simulink model "bldc_cImpl"  (R2018a)
settings: Solver=FixedStepDiscrete  StartTime=0.0  StopTime=5  FixedStep=Ts  RelTol=1e-3  EnableMultiTasking=on
undefined symbols (not defined in the file): fsw, Imax, Ki_id, Ki_iq, Kp_id, Kp_iq, Ld, p, Pmax, psim, sigbuilder_block, Tmax, Ts, Tsi, V1, Vnom, wbase
libraries: nesl_utility x12, fl_lib x11, pe_lib x5, pePwmGenerator x3, simulink_extras x1
Description:
  | IPMSM Torque Control in an Axle-Drive EV
  | 
  | Copyright 2017 The MathWorks, Inc.
settings Model: Creator=The MathWorks, Inc.  LastModifiedBy=Acer
settings SolverCC: AutoInsertRateTranBlk=on
settings DataIOCC: MaxDataPoints=510000  SignalLoggingName=logsout_pe_ipmsm_torque_control_ev_axle
settings OptimizationCC: LifeSpan=inf
settings DebuggingCC: UnderspecifiedInitializationDetection=Classic  MergeDetectMultiDrivingBlocksExec=none  SFUnexpectedBacktrackingDiag=warning  SFNoUnconditionalDefaultTransitionDiag=warning  SFExecutionAtInitializationDiag=none
settings CodeAppCC: StateflowObjectComments=on
settings GRTTargetCC: TargetLangStandard=C89/C90 (ANSI)  GeneratePreprocessorConditionals=Disable all
settings ConfigComp: CovMetricSettings=dw  CovHtmlReporting=on  CovSaveCumulativeToWorkspaceVar=on  CovSaveSingleToWorkspaceVar=on  CovExternalEMLEnable=off
settings SimscapeCC: SimscapeNormalizeSystem=off  SimscapeLogType=all  SimscapeLogSimulationStatistics=on  SimscapeLogName=simlog_pe_ipmsm_torque_control_ev_axle  SimscapeLogDataHistory=510000

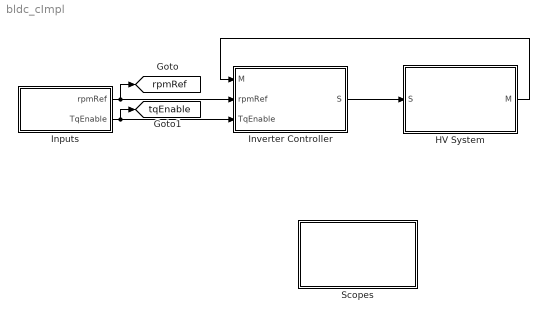
== system bldc_cImpl ==
  HV System : Subsystem
  Inputs : Subsystem  Tag=STV Subsys  LoadFcn=sigbuilder_block('load');  StartFcn=sigbuilder_block('start');  StopFcn=sigbuilder_block('stop');  ClipboardFcn=sigbuilder_block('clipboard');  mask(Sigbuilder block){tuvar=[0:10]}
      mask help: Simulink:masks:SigbuilderBlock_MD
      mask init:
      | if ~strcmp(get_param(bdroot(gcbh),'SimulationStatus'),'stopped') tuvar = sigbuilder_block('maskInit'); end
      settings: CopyFcn=sigbuilder_block('copy');  DeleteFcn=sigbuilder_block('delete');  ModelCloseFcn=sigbuilder_block('modelClose');  PreSaveFcn=sigbuilder_block('preSave');  PauseFcn=sigbuilder_block('pause');  ContinueFcn=sigbuilder_block('continue');  NameChangeFcn=sigbuilder_block('namechange');  OpenFcn=sigbuilder_block('open',[627 127.5 1012.5 512.25 ]);  CloseFcn=sigbuilder_block('close');
      mask Display: plot(0, 0, 100, 100,[2, 2, 32, 32, 2], [68, 8, 8, 68, 68],[32, 2], [38, 38], [32, 19, 2],[53, 60, 44], [32, 17, 17, 2],[16, 16, 31, 31]);txt = getActiveGroup(gcbh);text(2, 100, txt,'verticalAlignment', 'top');
  Inverter Controller : Subsystem
  Scopes : Subsystem
  tag scope: rpmRef=global, tqEnable=global
  wires:
  Inverter Controller/1(S) -> HV System/1(S)
  HV System/1(M) -> Inverter Controller/1(M)
  Inputs/1(rpmRef) -> Inverter Controller/2(rpmRef), [rpmRef]
  Inputs/2(TqEnable) -> [tqEnable], Inverter Controller/3(TqEnable)

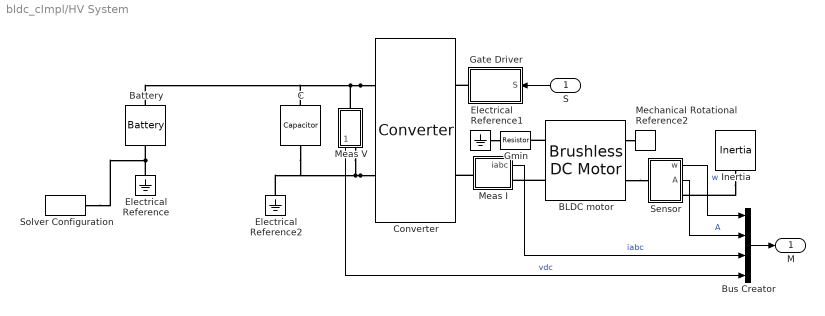
== system bldc_cImpl/HV System ==
  S : Inport
  BLDC motor : pe_lib/Machines/Permanent Magnet Rotor/Brushless DC Motor  rotor_param=1  pm_flux_linkage=psim Wb  theta_constant=pi / 12 rad  emf_max=9.6 V  DphiDtheta_tab=[0, -.1528, -.1528, .1528, .1528, 0] Wb/rad  back_emf_tab=[0, -9.6, -9.6, 9.6, 9.6, 0] V  rotor_angle_tab=[0, 7.5, 22.5, 37.5, 52.5, 60] deg  w_meas=600 rpm  nPolePairs=p  stator_param=1  Ld=Ld H  Lq=Lq H  L0=L0 H  Ls=0.0002 H  Lm=0 H  Ms=0.00002 H  Rs=Rs Ohm  zero_sequence=pe.enum.park.zerosequence.exclude  J=0 kg*m^2  lam=0 N*m/(rad/s)  axes_param=1  i_d_specify=off  i_d_priority=None  i_d=0 A  i_d_nominal_specify=off  i_d_nominal_unit=A  i_d_nominal_value=1  i_q_specify=off  i_q_priority=None  i_q=0 A  i_q_nominal_specify=off  i_q_nominal_unit=A  i_q_nominal_value=1  torque_specify=off  torque_priority=None  torque=0 N*m  torque_nominal_specify=off  torque_nominal_unit=N*m  torque_nominal_value=1  angular_velocity_specify=on  angular_velocity_priority=High  angular_velocity=0 rpm  angular_velocity_nominal_specify=off  angular_velocity_nominal_unit=rpm  angular_velocity_nominal_value=1  angular_position_specify=off  angular_position_priority=High  angular_position=0 deg  angular_position_nominal_specify=off  angular_position_nominal_unit=deg  angular_position_nominal_value=1
      settings: SourceProductName=Simscape Power Systems  SourceProductBaseCode=PS
  Battery : pe_lib/Sources/Battery  Vnom=Vnom V  R1=0.001 Ohm  prm_AH=1  AH=15000 hr*A  V1=V1 V  AH1=10000 hr*A  prm_R2=1  R2=2000 Ohm  prm_dyn=1  Rp1=0.005 Ohm  tau1=30 s  Rp2=0.005 Ohm  tau2=30 s  prm_fade=1  N_fade=100  AH_fade=45 hr*A  R1_fade=2.02 Ohm  V1_fade=10.35 V  i_specify=off  i_priority=None  i=0 A  i_nominal_specify=off  i_nominal_unit=A  i_nominal_value=1  v_specify=off  v_priority=None  v=0 V  v_nominal_specify=off  v_nominal_unit=V  v_nominal_value=1  charge_specify=on  charge_priority=High  charge=14000 hr*A  charge_nominal_specify=off  charge_nominal_unit=hr*A  charge_nominal_value=1  num_cycles_specify=off  num_cycles_priority=High  num_cycles=0  num_cycles_nominal_specify=off  num_cycles_nominal_unit=1  num_cycles_nominal_value=1  thermal_mass=30000 J/K  Tmeas=298.15 K  Vnom_T2=12 V  R1_T2=2.2 Ohm  V1_T2=11.4 V  R2_T2=2200 Ohm  Rp1_T2=0.005 Ohm  tau1_T2=30 s  Rp2_T2=0.005 Ohm  tau2_T2=30 s  Tmeas2=273.15 K  temperature_specify=off  temperature_priority=High  temperature=298.15 K  temperature_nominal_specify=off  temperature_nominal_unit=K  temperature_nominal_value=1
      settings: SourceProductName=Simscape Power Systems  SourceProductBaseCode=PS
  Bus Creator : BusCreator  Inputs=4
  C : fl_lib/Electrical/Electrical Elements/Capacitor  c=Cdc F  r=1e-6 Ohm  g=0 1/Ohm  i_specify=off  i_priority=None  i=0 A  i_nominal_specify=off  i_nominal_unit=A  i_nominal_value=1  v_specify=off  v_priority=None  v=0 V  v_nominal_specify=off  v_nominal_unit=V  v_nominal_value=1  vc_specify=off  vc_priority=High  vc=0 V  vc_nominal_specify=off  vc_nominal_unit=V  vc_nominal_value=1
      settings: SourceProductName=Foundation Library
  Converter : pe_lib/Semiconductors/Converter  device_type=3  Vf=0.8 V  Ron=0.001 Ohm  Rds=0.001 Ohm  Goff=1e-5 1/Ohm  Vth=0.5 V  Vgt=1 V  Vgt_off=-1 V  Ih=1 A  diode_param=2  diode_Vf=0.8 V  diode_Ron=0.001 Ohm  diode_Goff=1e-5 1/Ohm  diode_C=50 nF  diode_iRM=-235 A  diode_iF=300 A  diode_idot=-50 A/us  diode_trr_param=1  diode_trr_factor=3  diode_trr=15 us  diode_Qrr=1.5e+3 s*uA  snubber_type=0  Rs=0.1 Ohm  Cs=1e-7 F
      settings: SourceProductName=Simscape Power Systems  SourceProductBaseCode=PS
  Electrical Reference : fl_lib/Electrical/Electrical Elements/Electrical Reference
      settings: SourceProductName=Foundation Library
  Electrical Reference1 : fl_lib/Electrical/Electrical Elements/Electrical Reference
      settings: SourceProductName=Foundation Library
  Electrical Reference2 : fl_lib/Electrical/Electrical Elements/Electrical Reference
      settings: SourceProductName=Foundation Library
  Gate Driver : Subsystem
  Gmin : fl_lib/Electrical/Electrical Elements/Resistor  R=1e9 Ohm  i_specify=off  i_priority=High  i=0 A  i_nominal_specify=off  i_nominal_unit=A  i_nominal_value=1  v_specify=off  v_priority=High  v=0 V  v_nominal_specify=off  v_nominal_unit=V  v_nominal_value=1
      settings: SourceProductName=Foundation Library
  Inertia : fl_lib/Mechanical/Rotational Elements/Inertia  inertia=Jm kg*m^2  w_specify=off  w_priority=High  w=0 rad/s  w_nominal_specify=off  w_nominal_unit=rad/s  w_nominal_value=1  t_specify=off  t_priority=None  t=0 N*m  t_nominal_specify=off  t_nominal_unit=N*m  t_nominal_value=1
      settings: SourceProductName=Foundation Library
  Meas I : Subsystem
      mask Display: %disp('iABC');
  Meas V : Subsystem
  Mechanical Rotational Reference2 : fl_lib/Mechanical/Rotational Elements/Mechanical Rotational Reference
      settings: SourceProductName=Foundation Library
  Sensor : Subsystem
  Solver Configuration : nesl_utility/Solver Configuration  PhysicalDomain=network_engine_domain  SubClassName=solver  LeftPortType=input  RightPortType=generic  Tones=[]  Harmonics=[]  SimulateNoise=off  Profile=off  UseLocalSampling=off  EnableSwitchedLinearOptims=on  FrequencyDomain=off  UseCCode=off  RelTol=0.001  AbsTol=1e-06  MinStep=1e-09  ToWorkspace=off  RevertToSquareIcSolve=off  NumHomotopyIterations=100  PhasorMode=off  PhasorModeNumHarmonics=1  DoDC=off  ResidualTolerance=1e-9  UseLocalSolver=on  LocalSolverChoice=NE_BACKWARD_EULER_ADVANCER  LocalSolverSampleTime=Ts  DoFixedCost=on  MaxNonlinIter=4  MaxModeIter=2  LinearAlgebra=Sparse  EquationFormulation=NE_TIME_EF  DelaysMemoryBudget=1024  AutomaticFiltering=on  FilteringTimeConstant=0.001
  M : Outport
  wires:
  Meas V/1(Vdc) -> Bus Creator/4  "vdc"
  Sensor/2(A) -> Bus Creator/2  "A"
  Bus Creator/1 -> M/1
  Sensor/1(w) -> Bus Creator/1  "w"
  Meas I/1(iabc) -> Bus Creator/3  "iabc"
  S/1 -> Gate Driver/1(S)
  connections:
  Converter/RConn2 -- Electrical Reference2/LConn1 -- C/RConn1 -- Meas V/RConn1
  Converter/RConn1 -- Battery/LConn1 -- C/LConn1 -- Meas V/LConn1
  Inertia/LConn1 -- Sensor/RConn1
  BLDC motor/RConn2 -- Mechanical Rotational Reference2/LConn1
  BLDC motor/LConn1 -- Meas I/RConn1
  Gate Driver/RConn1 -- Converter/LConn1
  Meas I/LConn1 -- Converter/LConn2
  Electrical Reference1/LConn1 -- Gmin/LConn1
  BLDC motor/RConn1 -- Sensor/LConn1
  BLDC motor/LConn2 -- Gmin/RConn1
  Battery/RConn1 -- Electrical Reference/LConn1 -- Solver Configuration/RConn1

== system bldc_cImpl/Inputs ==
  Demux : Demux  Tag=STV Demux  Outputs=2
  FromWs : FromWorkspace  Tag=STV FromWs  VariableName=tuvar  SampleTime=0
      SigBuilderData=|
      | common.afterFinalStr = 'Extrapolate'
      | common.sampleTime = 0
      | dataSet.timeRange = [0 15]
      | dataSet.name = 'Default'
      | sbobj.Groups.Name = 'Default'
      | sbobj.Groups.Signals(1).Name = 'rpmRef'
      | sbobj.Groups.Signals(1).XData = [0 0.7 0.7 2 2 3.12 3.5 4 4.5 15]
      | sbobj.Groups.Signals(1).YData = [0 0 1500 1500 0 0 -1000 -1000 0 0]
      | sbobj.Groups.Signals(2).Name = 'TqEnable'
      | sbobj.Groups.Signals(2).XData = [0 15]
      | sbobj.Groups.Signals(2).YData = [1 1]
      | sbobj.Groups.TimeRange = [0 15]
  rpmRef : Outport  Tag=STV Outport
  TqEnable : Outport  Tag=STV Outport  Port=2
  wires:
  FromWs/1 -> Demux/1
  Demux/1 -> rpmRef/1
  Demux/2 -> TqEnable/1

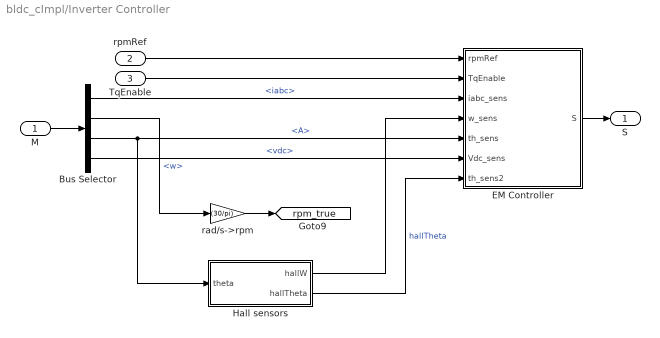
== system bldc_cImpl/Inverter Controller ==
  M : Inport
  rpmRef : Inport  Port=2
  TqEnable : Inport  Port=3
  Bus Selector : BusSelector  OutputSignals=iabc,w,A,vdc
  EM Controller : Subsystem
  Hall sensors : Subsystem
  rad/s->rpm : Gain  Gain=(30/pi)
  S : Outport
  tag scope: rpm_true=global
  wires:
  M/1 -> Bus Selector/1
  rpmRef/1 -> EM Controller/1(rpmRef)
  Bus Selector/1 -> EM Controller/3(iabc_sens)  "<iabc>"
  Bus Selector/3 -> Hall sensors/1(theta), EM Controller/5(th_sens)  "<A>"
  Bus Selector/4 -> EM Controller/6(Vdc_sens)  "<vdc>"
  EM Controller/1(S) -> S/1
  TqEnable/1 -> EM Controller/2(TqEnable)
  Bus Selector/2 -> rad/s->rpm/1  "<w>"
  Hall sensors/1(hallW) -> EM Controller/4(w_sens)
  Hall sensors/2(hallTheta) -> EM Controller/7(th_sens2)  "hallTheta"
  rad/s->rpm/1 -> [rpm_true]

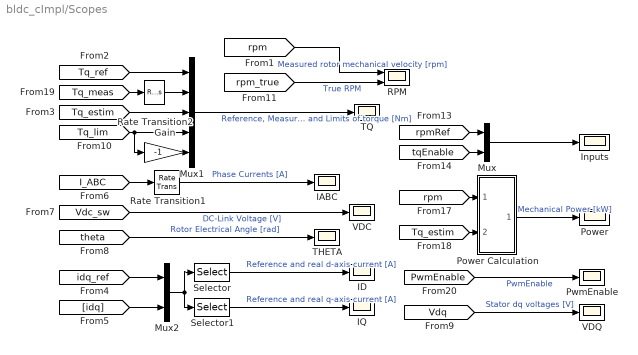
== system bldc_cImpl/Scopes ==
  Gain : Gain  Gain=-1
  IABC : Scope
  ID : Scope
  IQ : Scope
  Inputs : Scope
  Mux : Mux  Inputs=2
  Mux1 : Mux  Inputs=5
  Mux2 : Mux  Inputs=2
  Power : Scope
  Power Calculation : Subsystem
  PwmEnable : Scope
  RPM : Scope  NumInputPorts=2
  Rate Transition1 : RateTransition  OutPortSampleTime=1e-4
  Rate Transition2 : RateTransition
  Selector : Selector  InputPortWidth=4  IndexOptions=Index vector (dialog)  Indices=[1 3]  OutputSizes=1
  Selector1 : Selector  InputPortWidth=4  IndexOptions=Index vector (dialog)  Indices=[2 4]  OutputSizes=1
  THETA : Scope
  TQ : Scope
  VDC : Scope
  VDQ : Scope
  wires:
  Power Calculation/1(Power) -> Power/1  "Mechanical Power [kW]"
  Gain/1 -> Mux1/5
  [idq] -> Mux2/2
  [Tq_meas] -> Rate Transition2/1
  [Tq_estim] -> Mux1/3
  [rpm] -> Power Calculation/1(rpm)
  [Tq_estim] -> Power Calculation/2(Tq)
  [idq_ref] -> Mux2/1
  Mux1/1 -> TQ/1  "Reference, Measured, Estim and Limits of torque [Nm]"
  [Vdq] -> VDQ/1  "Stator dq voltages [V]"
  [I_ABC] -> Rate Transition1/1
  [Tq_ref] -> Mux1/1
  [Tq_lim] -> Gain/1, Mux1/4
  [PwmEnable] -> PwmEnable/1  "PwmEnable"
  Rate Transition2/1 -> Mux1/2
  [theta] -> THETA/1  "Rotor Electrical Angle [rad]"
  Selector/1 -> ID/1  "Reference and real d-axis current [A]"
  Mux2/1 -> Selector1/1, Selector/1
  Mux/1 -> Inputs/1
  Selector1/1 -> IQ/1  "Reference and real q-axis current [A]"
  [tqEnable] -> Mux/2
  [rpmRef] -> Mux/1
  Rate Transition1/1 -> IABC/1  "Phase Currents [A]"
  [rpm] -> RPM/1  "Measured rotor mechanical velocity [rpm]"
  [Vdc_sw] -> VDC/1  "DC-Link Voltage [V]"
  [rpm_true] -> RPM/2  "True RPM"

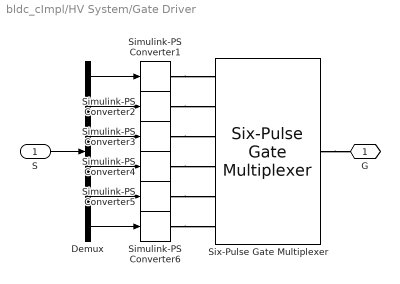
== system bldc_cImpl/HV System/Gate Driver ==
  S : Inport
  Demux : Demux  Outputs=6
  Simulink-PS Converter{1..6} (6 alike) : nesl_utility/Simulink-PS Converter  PhysicalDomain=network_engine_domain  SubClassName=ps_input  LeftPortType=input  RightPortType=output  PseudoPeriodic=off  Frequencies=[]  NoiseDistribution=none  NoiseParameters=[]  Unit=1  AffineConversion=off  FilteringAndDerivatives=zero  SimscapeFilterOrder=1  InputFilterTimeConstant=0.001  UdotUserProvided=1
  Six-Pulse Gate Multiplexer : pe_lib/Semiconductors/Six-Pulse Gate Multiplexer  R=0 Ohm
      settings: SourceProductName=Simscape Power Systems  SourceProductBaseCode=PS
  G : PMIOPort  Side=Right
  wires:
  Demux/1 -> Simulink-PS Converter1/1
  S/1 -> Demux/1
  Demux/4 -> Simulink-PS Converter4/1
  Demux/2 -> Simulink-PS Converter2/1
  Demux/3 -> Simulink-PS Converter3/1
  Demux/5 -> Simulink-PS Converter5/1
  Demux/6 -> Simulink-PS Converter6/1
  connections:
  Six-Pulse Gate Multiplexer/RConn1 -- G/RConn1
  Simulink-PS Converter1/RConn1 -- Six-Pulse Gate Multiplexer/LConn1
  Simulink-PS Converter3/RConn1 -- Six-Pulse Gate Multiplexer/LConn3
  Simulink-PS Converter5/RConn1 -- Six-Pulse Gate Multiplexer/LConn5
  Simulink-PS Converter6/RConn1 -- Six-Pulse Gate Multiplexer/LConn6
  Simulink-PS Converter4/RConn1 -- Six-Pulse Gate Multiplexer/LConn4
  Simulink-PS Converter2/RConn1 -- Six-Pulse Gate Multiplexer/LConn2

== system bldc_cImpl/HV System/Meas I ==
  Current Sensor : pe_lib/Sensors/Current Sensor
      settings: SourceProductName=Simscape Power Systems  SourceProductBaseCode=PS
  PS-Simulink Converter : nesl_utility/PS-Simulink Converter  PhysicalDomain=network_engine_domain  SubClassName=ps_output  LeftPortType=input  RightPortType=output  PseudoPeriodic=off  Frequencies=[]  Unit=A  AffineConversion=off
  1 : PMIOPort  Side=Left
  2 : PMIOPort  Port=2  Side=Right
  iabc : Outport
  tag scope: I_ABC=global
  wires:
  PS-Simulink Converter/1 -> [I_ABC], iabc/1
  connections:
  1/RConn1 -- Current Sensor/LConn1
  2/RConn1 -- Current Sensor/RConn2
  Current Sensor/RConn1 -- PS-Simulink Converter/LConn1

== system bldc_cImpl/HV System/Meas V ==
  PS-Simulink Converter4 : nesl_utility/PS-Simulink Converter  PhysicalDomain=network_engine_domain  SubClassName=ps_output  LeftPortType=input  RightPortType=output  PseudoPeriodic=off  Frequencies=[]  Unit=V  AffineConversion=off
  Voltage Sensor : fl_lib/Electrical/Electrical Sensors/Voltage Sensor
      settings: SourceProductName=Foundation Library
  - : PMIOPort  Side=Right
  + : PMIOPort  Port=2  Side=Left
  Vdc : Outport
  wires:
  PS-Simulink Converter4/1 -> Vdc/1
  connections:
  PS-Simulink Converter4/LConn1 -- Voltage Sensor/RConn1
  Voltage Sensor/LConn1 -- +/RConn1
  Voltage Sensor/RConn2 -- -/RConn1

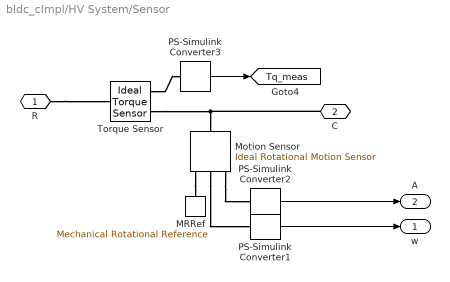
== system bldc_cImpl/HV System/Sensor ==
  MRRef : fl_lib/Mechanical/Rotational Elements/Mechanical Rotational Reference
      settings: SourceProductName=Foundation Library
  Motion Sensor : fl_lib/Mechanical/Mechanical Sensors/Ideal Rotational Motion Sensor  offset=0 deg
      settings: SourceProductName=Foundation Library
  PS-Simulink Converter1 : nesl_utility/PS-Simulink Converter  PhysicalDomain=network_engine_domain  SubClassName=ps_output  LeftPortType=input  RightPortType=output  PseudoPeriodic=off  Frequencies=[]  Unit=rad/s  AffineConversion=off
  PS-Simulink Converter2 : nesl_utility/PS-Simulink Converter  PhysicalDomain=network_engine_domain  SubClassName=ps_output  LeftPortType=input  RightPortType=output  PseudoPeriodic=off  Frequencies=[]  Unit=rad  AffineConversion=off
  PS-Simulink Converter3 : nesl_utility/PS-Simulink Converter  PhysicalDomain=network_engine_domain  SubClassName=ps_output  LeftPortType=input  RightPortType=output  PseudoPeriodic=off  Frequencies=[]  Unit=N*m  AffineConversion=off
  Torque Sensor : fl_lib/Mechanical/Mechanical Sensors/Ideal Torque Sensor
      settings: SourceProductName=Foundation Library
  R : PMIOPort  Side=Left
  C : PMIOPort  Port=2  Side=Right
  w : Outport
  A : Outport  Port=2
  tag scope: Tq_meas=global
  wires:
  PS-Simulink Converter3/1 -> [Tq_meas]
  PS-Simulink Converter2/1 -> A/1
  PS-Simulink Converter1/1 -> w/1
  connections:
  Motion Sensor/RConn2 -- PS-Simulink Converter1/LConn1
  Motion Sensor/RConn1 -- MRRef/LConn1
  R/RConn1 -- Torque Sensor/LConn1
  Torque Sensor/RConn1 -- C/RConn1 -- Motion Sensor/LConn1
  Torque Sensor/RConn2 -- PS-Simulink Converter3/LConn1
  Motion Sensor/RConn3 -- PS-Simulink Converter2/LConn1

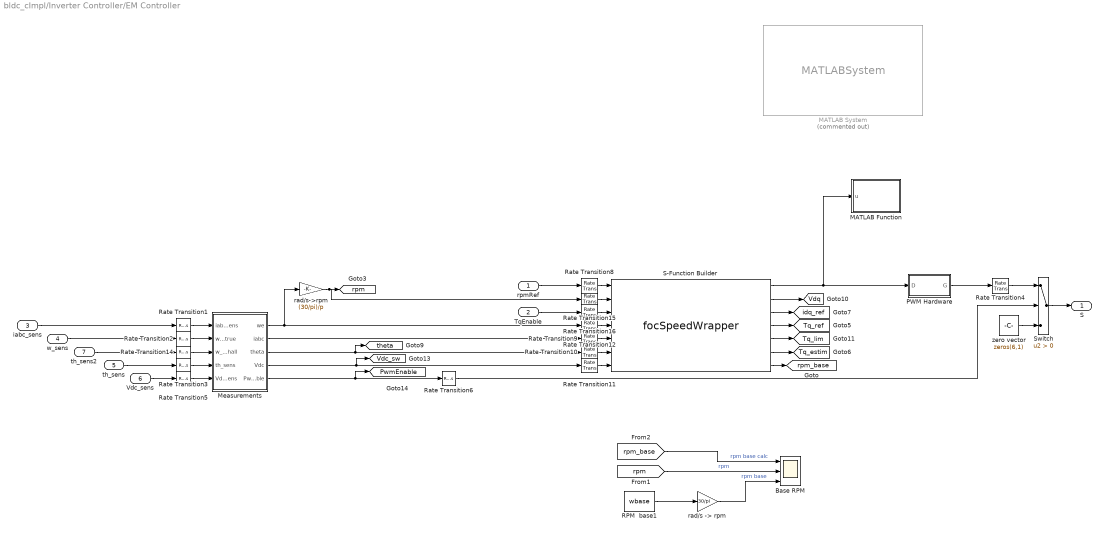
== system bldc_cImpl/Inverter Controller/EM Controller ==
  rpmRef : Inport
  TqEnable : Inport  Port=2
  iabc_sens : Inport  Port=3
  w_sens : Inport  Port=4
  th_sens : Inport  Port=5
  Vdc_sens : Inport  Port=6
  th_sens2 : Inport  Port=7
  Base RPM : Scope  NumInputPorts=3
  MATLAB Function : MATLAB Function  TreatAsAtomicUnit=on
  MATLAB System : MATLABSystem  Commented=on  System=FieldOrientedSpeedControl  T=Tsi  Vnom=Vnom  Pmax=Pmax  Tmax=Tmax  Imax=Imax  p=p  psim=psim  Rs=Rs  Ld=Ld  Lq=Lq  wBase=wbase  Kp_id=Kp_id  Ki_id=Ki_id  AntiWindUpD=1  Kp_iq=Kp_iq  Ki_iq=Ki_iq  AntiWindUpQ=1  Kp_speed=0.1  Ki_speed=0  AntiWindUpSpeed=1  SimulateUsing=Code generation
      mask Type: FieldOrientedSpeedControl
      mask Display:
      | disp('FieldOrientedSpeedControl');
      | port_label('input',1,'RpmRef');
      | port_label('input',2,'RpmMeas');
      | port_label('input',3,'TqEnable');
      | port_label('input',4,'we');
      | port_label('input',5,'iabc');
      | port_label('input',6,'theta_e');
      | port_label('input',7,'Vdc');
      | port_label('output',1,'Dabc');
      | port_label('output',2,'Vdq');
      | port_label('output',3,'idqRef');
      | port_label('output',4,'TqRefSat');
      | port_label('output',5,'TqLim');
      | port_label('output',6,'TqEst');
      | port_label('output',7,'rpm_base');
  Measurements : Subsystem
  PWM Hardware : Subsystem
  RPM  base1 : Constant  Value=wbase
  Rate Transition{1..3,5,8..12,14..16} (12 alike) : RateTransition  OutPortSampleTime=Tsi
  Rate Transition4 : RateTransition
  Rate Transition6 : RateTransition
  S-Function Builder : S-Function  InitFcn=try, set_param(gcb,'FunctionName','focSpeedWrapper'), end  FunctionName=focSpeedWrapper  Parameters=Tsi,Kp_id,Ki_id,Kp_iq,Ki_iq,0.1,0,p,Vnom,Pmax,Tmax,Imax,wbase,psim,Ld  SFunctionModules=focSpeedWrapper_wrapper PMSMCurrentController PMSMCurrentRef PMSMFOC SPWM transforms pid sat lowPassFilter focSpeed  SFunctionDeploymentMode=off  EnableBusSupport=off  mask(S-Function Builder){}
      mask help: Simulink:masks:SFunctionBuilder_MD
      mask init:
      | val = [[.9  0.75 0.75 1 1 .9 .9 1]',[1 1 0.75 0.75 .9 .9 1 .9]'];try , sys = get_param(gcb,'SfunBuilderFcnName');if isempty(sys), sys = get_param(gcb,'FunctionName'); end,catch, sys = get_param(gcb,'FunctionName'); end
      settings: CopyFcn=set_param(gcbh,'LinkStatus','none')  PreSaveFcn=try, set_param(gcb,'FunctionName','focSpeedWrapper'), end  OpenFcn=sfunctionwizard(gcbh)
      mask Display:
      | plot(val(:,1),val(:,2))
      | disp(sys)
      | port_label('input',1,'rpmRef')
      | port_label('input',2,'rpmMeas')
      | port_label('input',3,'tqEnable')
      | port_label('input',4,'w_sense')
      | port_label('input',5,'iabc_sense')
      | port_label('input',6,'th_sense')
      | port_label('input',7,'Vdc_sense')
      | port_label('output',1,'Dabc')
      | port_label('output',2,'Vdq')
      | port_label('output',3,'idqRef')
      | port_label('output',4,'TqRefSat')
      | port_label('output',5,'TqLim')
      | port_label('output',6,'TqEst')
      | port_label('output',7,'rpm_base')
  Switch : Switch  Criteria=u2 > Threshold
  "rad/s -> rpm" : Gain  Gain=30/pi
  rad/s->rpm : Gain  Gain=(30/pi)/p
  zero vector : Constant  Value=zeros(6,1)
  S : Outport
  tag scope: PwmEnable=global, Tq_estim=global, Tq_lim=global, Tq_ref=global, Vdc_sw=global, Vdq=global, idq_ref=global, rpm=global, rpm_base=global, theta=global
  wires:
  Measurements/5(PwmEnable) -> [PwmEnable], Rate Transition6/1
  Rate Transition3/1 -> Measurements/4(th_sens)
  Rate Transition6/1 -> Switch/2
  Vdc_sens/1 -> Rate Transition5/1
  Measurements/4(Vdc) -> [Vdc_sw], Rate Transition11/1
  Measurements/1(we) -> rad/s->rpm/1, Rate Transition12/1
  Rate Transition5/1 -> Measurements/5(Vdc_sens)
  Measurements/3(theta) -> [theta], Rate Transition10/1
  iabc_sens/1 -> Rate Transition1/1
  th_sens/1 -> Rate Transition3/1
  Rate Transition2/1 -> Measurements/2(w_sens_true)
  Rate Transition4/1 -> Switch/1
  Switch/1 -> S/1
  w_sens/1 -> Rate Transition2/1
  Rate Transition1/1 -> Measurements/1(iabc_sens)
  zero vector/1 -> Switch/3
  Measurements/2(iabc) -> Rate Transition9/1
  PWM Hardware/1(G) -> Rate Transition4/1
  Rate Transition11/1 -> S-Function Builder/7
  Rate Transition10/1 -> S-Function Builder/6
  S-Function Builder/1 -> MATLAB Function/1(u), PWM Hardware/1(D)
  Rate Transition8/1 -> S-Function Builder/1
  S-Function Builder/2 -> [Vdq]
  Rate Transition9/1 -> S-Function Builder/5
  Rate Transition12/1 -> S-Function Builder/4
  S-Function Builder/3 -> [idq_ref]
  S-Function Builder/4 -> [Tq_ref]
  S-Function Builder/5 -> [Tq_lim]
  S-Function Builder/6 -> [Tq_estim]
  [rpm] -> Base RPM/2  "rpm"
  [rpm_base] -> Base RPM/1  "rpm base calc"
  "rad/s -> rpm"/1 -> Base RPM/3  "rpm base"
  RPM  base1/1 -> "rad/s -> rpm"/1
  S-Function Builder/7 -> [rpm_base]
  rad/s->rpm/1 -> [rpm], Rate Transition15/1
  th_sens2/1 -> Rate Transition14/1
  Rate Transition15/1 -> S-Function Builder/2
  Rate Transition16/1 -> S-Function Builder/3
  Rate Transition14/1 -> Measurements/3(w_sens_hall)
  rpmRef/1 -> Rate Transition8/1
  TqEnable/1 -> Rate Transition16/1

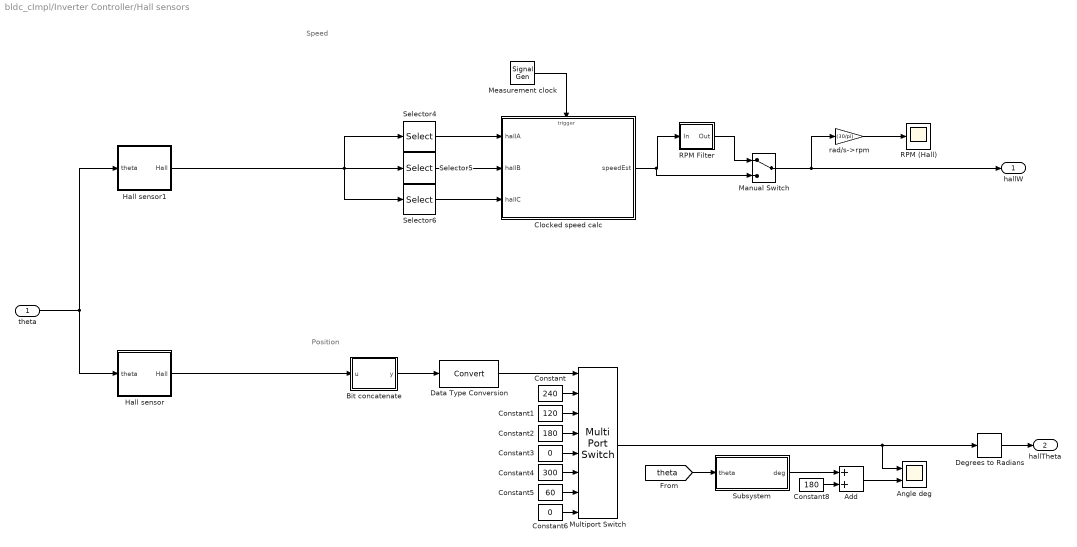
== system bldc_cImpl/Inverter Controller/Hall sensors ==
  note: Speed
  note: Position
  theta : Inport
  Add : Sum
  Angle deg : Scope  NumInputPorts=2
  Bit concatenate : Subsystem
  Clocked speed calc : Subsystem
  Constant : Constant  Value=240
  Constant1 : Constant  Value=120
  Constant2 : Constant  Value=180
  Constant3 : Constant  Value=0
  Constant4 : Constant  Value=300
  Constant5 : Constant  Value=60
  Constant6 : Constant  Value=0
  Constant8 : Constant  Value=180
  Data Type Conversion : DataTypeConversion
  Degrees to Radians : simulink_extras/Transformations/Degrees to Radians
  Hall sensor : Subsystem
  Hall sensor1 : Subsystem
  Manual Switch : ManualSwitch
  Measurement clock : SignalGenerator  WaveForm=square  Frequency=10000
  Multiport Switch : MultiPortSwitch  Inputs=6  DataPortForDefault=Additional data port
  RPM (Hall) : Scope
  RPM Filter : Subsystem  mask(Discrete first-order filter (Low-pass)){T=1, Ts=Tsi}
      mask prompts: T "Time constant (s):"; Ts "Sample time (s):"
      mask help: This block implements a discrete low-pass filter. To calculate the coefficients, the block discretises a continuous low-pass filter using the Tustin method.
      mask init:
      | num = [ Ts/(2*T + Ts), Ts/(2*T + Ts)];
      | den = [ 1, -(2*T - Ts)/(2*T + Ts)];
  Selector4 : Selector  InputPortWidth=3  IndexOptions=Index vector (dialog)  Indices=1  OutputSizes=1
  Selector5 : Selector  InputPortWidth=3  IndexOptions=Index vector (dialog)  Indices=2  OutputSizes=1
  Selector6 : Selector  InputPortWidth=3  IndexOptions=Index vector (dialog)  Indices=3  OutputSizes=1
  Subsystem : Subsystem
  rad/s->rpm : Gain  Gain=(30/pi)
  hallW : Outport
  hallTheta : Outport  Port=2
  wires:
  theta/1 -> Hall sensor1/1(theta), Hall sensor/1(theta)
  Constant8/1 -> Add/2
  Add/1 -> Angle deg/2
  [theta] -> Subsystem/1(theta)
  Subsystem/1(deg) -> Add/1
  Constant2/1 -> Multiport Switch/4
  Hall sensor1/1(Hall) -> Selector6/1, Selector5/1, Selector4/1
  Constant5/1 -> Multiport Switch/7
  Constant3/1 -> Multiport Switch/5
  Constant4/1 -> Multiport Switch/6
  Constant/1 -> Multiport Switch/2
  Constant6/1 -> Multiport Switch/8
  Bit concatenate/1(y) -> Data Type Conversion/1
  Constant1/1 -> Multiport Switch/3
  Data Type Conversion/1 -> Multiport Switch/1
  Multiport Switch/1 -> Degrees to Radians/1, Angle deg/1
  Selector6/1 -> Clocked speed calc/3(hallC)
  Selector5/1 -> Clocked speed calc/2(hallB)
  Selector4/1 -> Clocked speed calc/1(hallA)
  Measurement clock/1 -> Clocked speed calc/Trigger
  Clocked speed calc/1(speedEst) -> Manual Switch/2, RPM Filter/1(In)
  rad/s->rpm/1 -> RPM (Hall)/1
  Manual Switch/1 -> hallW/1, rad/s->rpm/1
  RPM Filter/1(Out) -> Manual Switch/1
  Degrees to Radians/1 -> hallTheta/1
  Hall sensor/1(Hall) -> Bit concatenate/1(u)

== system bldc_cImpl/Scopes/Power Calculation ==
  rpm : Inport
  Tq : Inport  Port=2
  Gain3 : Gain  Gain=pi/30
  Gain4 : Gain  Gain=1/1000
  Product2 : Product
  Power : Outport
  wires:
  rpm/1 -> Gain3/1
  Gain4/1 -> Power/1
  Product2/1 -> Gain4/1
  Tq/1 -> Product2/2
  Gain3/1 -> Product2/1

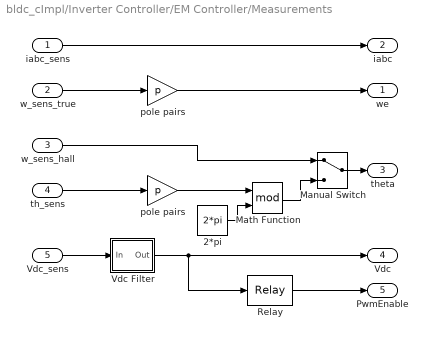
== system bldc_cImpl/Inverter Controller/EM Controller/Measurements ==
  iabc_sens : Inport
  w_sens_true : Inport  Port=2
  w_sens_hall : Inport  Port=3
  th_sens : Inport  Port=4
  Vdc_sens : Inport  Port=5
  2*pi : Constant  Value=2*pi  SampleTime=Tsi
  Manual Switch : ManualSwitch
  Math Function : Math  Operator=mod  SaturateOnIntegerOverflow=on
  Relay : Relay  OnSwitchValue=V1/2  OffSwitchValue=V1/4
  Vdc Filter : Subsystem  mask(Discrete first-order filter (Low-pass)){T=0.01, Ts=Tsi}
      mask prompts: T "Time constant (s):"; Ts "Sample time (s):"
      mask help: This block implements a discrete low-pass filter. To calculate the coefficients, the block discretises a continuous low-pass filter using the Tustin method.
      mask init:
      | num = [ Ts/(2*T + Ts), Ts/(2*T + Ts)];
      | den = [ 1, -(2*T - Ts)/(2*T + Ts)];
  pole pairs : Gain  Gain=p
  "pole pairs " : Gain  Gain=p
  we : Outport
  iabc : Outport  Port=2
  theta : Outport  Port=3
  Vdc : Outport  Port=4
  PwmEnable : Outport  Port=5
  wires:
  pole pairs/1 -> we/1
  th_sens/1 -> "pole pairs "/1
  w_sens_true/1 -> pole pairs/1
  iabc_sens/1 -> iabc/1
  2*pi/1 -> Math Function/2
  "pole pairs "/1 -> Math Function/1
  Vdc_sens/1 -> Vdc Filter/1(In)
  Relay/1 -> PwmEnable/1
  Vdc Filter/1(Out) -> Relay/1, Vdc/1
  Manual Switch/1 -> theta/1
  Math Function/1 -> Manual Switch/2
  w_sens_hall/1 -> Manual Switch/1

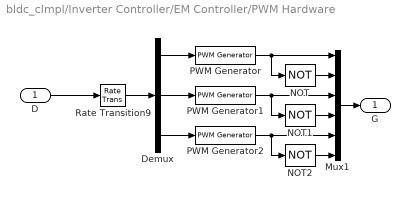
== system bldc_cImpl/Inverter Controller/EM Controller/PWM Hardware ==
  D : Inport
  Demux : Demux  Outputs=3
  Mux1 : Mux  Inputs=6
  NOT : Logic  Operator=NOT  IconShape=distinctive  AllPortsSameDT=off  OutDataTypeStr=boolean
  NOT1 : Logic  Operator=NOT  IconShape=distinctive  AllPortsSameDT=off  OutDataTypeStr=boolean
  NOT2 : Logic  Operator=NOT  IconShape=distinctive  AllPortsSameDT=off  OutDataTypeStr=boolean
  PWM Generator : pePwmGenerator/PWM Generator  CarrCount=Up  Tper=1/fsw  Ts=Ts
  PWM Generator1 : pePwmGenerator/PWM Generator  CarrCount=Up  Tper=1/fsw  Ts=Ts
  PWM Generator2 : pePwmGenerator/PWM Generator  CarrCount=Up  Tper=1/fsw  Ts=Ts
  Rate Transition9 : RateTransition
  G : Outport
  wires:
  PWM Generator/1 -> NOT/1, Mux1/1
  Demux/1 -> PWM Generator/1
  NOT1/1 -> Mux1/4
  PWM Generator1/1 -> Mux1/3, NOT1/1
  NOT2/1 -> Mux1/6
  NOT/1 -> Mux1/2
  PWM Generator2/1 -> Mux1/5, NOT2/1
  Demux/2 -> PWM Generator1/1
  Demux/3 -> PWM Generator2/1
  Mux1/1 -> G/1
  D/1 -> Rate Transition9/1
  Rate Transition9/1 -> Demux/1

== system bldc_cImpl/Inverter Controller/Hall sensors/Bit concatenate ==
  u : Inport
  Gain : Gain  Gain=[4 2 1]  Multiplication=Matrix(K*u)
  Sum of Elements : Sum  Inputs=+
  y : Outport
  wires:
  u/1 -> Gain/1
  Gain/1 -> Sum of Elements/1
  Sum of Elements/1 -> y/1

== system bldc_cImpl/Inverter Controller/Hall sensors/Clocked speed calc ==
  hallA : Inport
  hallB : Inport  Port=2
  hallC : Inport  Port=3
  Trigger : TriggerPort  VariantControl=Variant  PortDimensions=1
  MATLAB Function : MATLAB Function  TreatAsAtomicUnit=on
  speedEst : Outport
  wires:
  MATLAB Function/1(w) -> speedEst/1
  hallB/1 -> MATLAB Function/2(hallB)
  hallA/1 -> MATLAB Function/1(hallA)
  hallC/1 -> MATLAB Function/3(hallC)

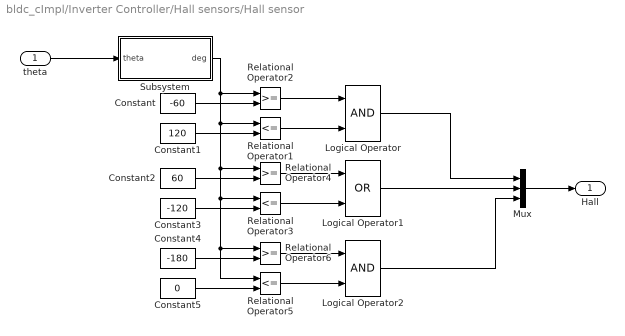
== system bldc_cImpl/Inverter Controller/Hall sensors/Hall sensor ==
  theta : Inport
  Constant : Constant  Value=-60
  Constant1 : Constant  Value=120
  Constant2 : Constant  Value=60
  Constant3 : Constant  Value=-120
  Constant4 : Constant  Value=-180
  Constant5 : Constant  Value=0
  Logical Operator : Logic  AllPortsSameDT=off  OutDataTypeStr=boolean
  Logical Operator1 : Logic  Operator=OR  AllPortsSameDT=off  OutDataTypeStr=boolean
  Logical Operator2 : Logic  AllPortsSameDT=off  OutDataTypeStr=boolean
  Mux : Mux  Inputs=3
  Relational Operator1 : RelationalOperator  Operator=<=  RndMeth=Nearest  InputSameDT=on
  Relational Operator2 : RelationalOperator  RndMeth=Nearest  InputSameDT=on
  Relational Operator3 : RelationalOperator  Operator=<=  RndMeth=Nearest  InputSameDT=on
  Relational Operator4 : RelationalOperator  RndMeth=Nearest  InputSameDT=on
  Relational Operator5 : RelationalOperator  Operator=<=  RndMeth=Nearest  InputSameDT=on
  Relational Operator6 : RelationalOperator  RndMeth=Nearest  InputSameDT=on
  Subsystem : Subsystem
  Hall : Outport
  wires:
  Constant3/1 -> Relational Operator3/2
  Logical Operator2/1 -> Mux/3
  Logical Operator1/1 -> Mux/2
  Logical Operator/1 -> Mux/1
  Relational Operator5/1 -> Logical Operator2/2
  Relational Operator6/1 -> Logical Operator2/1
  Constant4/1 -> Relational Operator6/2
  Constant5/1 -> Relational Operator5/2
  Relational Operator3/1 -> Logical Operator1/2
  Mux/1 -> Hall/1
  Relational Operator2/1 -> Logical Operator/1
  Relational Operator1/1 -> Logical Operator/2
  Subsystem/1(deg) -> Relational Operator4/1, Relational Operator3/1, Relational Operator5/1, Relational Operator6/1, Relational Operator1/1, Relational Operator2/1
  Constant/1 -> Relational Operator2/2
  Relational Operator4/1 -> Logical Operator1/1
  Constant1/1 -> Relational Operator1/2
  Constant2/1 -> Relational Operator4/2
  theta/1 -> Subsystem/1(theta)

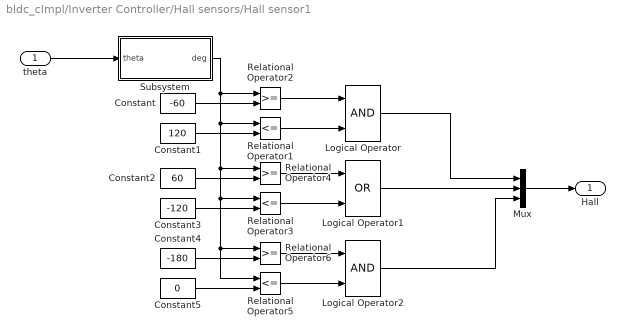
== system bldc_cImpl/Inverter Controller/Hall sensors/Hall sensor1 ==
  theta : Inport
  Constant : Constant  Value=-60
  Constant1 : Constant  Value=120
  Constant2 : Constant  Value=60
  Constant3 : Constant  Value=-120
  Constant4 : Constant  Value=-180
  Constant5 : Constant  Value=0
  Logical Operator : Logic  AllPortsSameDT=off  OutDataTypeStr=boolean
  Logical Operator1 : Logic  Operator=OR  AllPortsSameDT=off  OutDataTypeStr=boolean
  Logical Operator2 : Logic  AllPortsSameDT=off  OutDataTypeStr=boolean
  Mux : Mux  Inputs=3
  Relational Operator1 : RelationalOperator  Operator=<=  RndMeth=Nearest  InputSameDT=on
  Relational Operator2 : RelationalOperator  RndMeth=Nearest  InputSameDT=on
  Relational Operator3 : RelationalOperator  Operator=<=  RndMeth=Nearest  InputSameDT=on
  Relational Operator4 : RelationalOperator  RndMeth=Nearest  InputSameDT=on
  Relational Operator5 : RelationalOperator  Operator=<=  RndMeth=Nearest  InputSameDT=on
  Relational Operator6 : RelationalOperator  RndMeth=Nearest  InputSameDT=on
  Subsystem : Subsystem
  Hall : Outport
  wires:
  Constant3/1 -> Relational Operator3/2
  Logical Operator2/1 -> Mux/3
  Logical Operator1/1 -> Mux/2
  Logical Operator/1 -> Mux/1
  Relational Operator5/1 -> Logical Operator2/2
  Relational Operator6/1 -> Logical Operator2/1
  Constant4/1 -> Relational Operator6/2
  Constant5/1 -> Relational Operator5/2
  Relational Operator3/1 -> Logical Operator1/2
  Mux/1 -> Hall/1
  Relational Operator2/1 -> Logical Operator/1
  Relational Operator1/1 -> Logical Operator/2
  Subsystem/1(deg) -> Relational Operator4/1, Relational Operator3/1, Relational Operator5/1, Relational Operator6/1, Relational Operator1/1, Relational Operator2/1
  Constant/1 -> Relational Operator2/2
  Relational Operator4/1 -> Logical Operator1/1
  Constant1/1 -> Relational Operator1/2
  Constant2/1 -> Relational Operator4/2
  theta/1 -> Subsystem/1(theta)

== system bldc_cImpl/Inverter Controller/Hall sensors/RPM Filter ==
  In : Inport
  Discrete Transfer Fcn : DiscreteTransferFcn  Numerator=num  Denominator=den
  Out : Outport
  wires:
  In/1 -> Discrete Transfer Fcn/1
  Discrete Transfer Fcn/1 -> Out/1

== system bldc_cImpl/Inverter Controller/Hall sensors/Subsystem ==
  theta : Inport
  Trigonometric Function : Trigonometry  Operator=sincos
  Trigonometric Function2 : Trigonometry  Operator=atan2
  mech->elec : Gain  Gain=p
  rad->deg : Gain  Gain=180/pi  SaturateOnIntegerOverflow=on  OutDataTypeStr=Inherit: Same as input  ParamDataTypeStr=Inherit: Same as input
  deg : Outport
  wires:
  Trigonometric Function2/1 -> rad->deg/1
  Trigonometric Function/1 -> Trigonometric Function2/1
  theta/1 -> mech->elec/1
  rad->deg/1 -> deg/1
  Trigonometric Function/2 -> Trigonometric Function2/2
  mech->elec/1 -> Trigonometric Function/1

== system bldc_cImpl/Inverter Controller/EM Controller/Measurements/Vdc Filter ==
  In : Inport
  Discrete Transfer Fcn : DiscreteTransferFcn  Numerator=num  Denominator=den
  Out : Outport
  wires:
  In/1 -> Discrete Transfer Fcn/1
  Discrete Transfer Fcn/1 -> Out/1

== system bldc_cImpl/Inverter Controller/Hall sensors/Hall sensor/Subsystem ==
  theta : Inport
  Trigonometric Function : Trigonometry  Operator=sincos
  Trigonometric Function2 : Trigonometry  Operator=atan2
  mech->elec : Gain  Gain=p
  rad->deg : Gain  Gain=180/pi  SaturateOnIntegerOverflow=on  OutDataTypeStr=Inherit: Same as input  ParamDataTypeStr=Inherit: Same as input
  deg : Outport
  wires:
  Trigonometric Function2/1 -> rad->deg/1
  Trigonometric Function/1 -> Trigonometric Function2/1
  theta/1 -> mech->elec/1
  rad->deg/1 -> deg/1
  Trigonometric Function/2 -> Trigonometric Function2/2
  mech->elec/1 -> Trigonometric Function/1

== system bldc_cImpl/Inverter Controller/Hall sensors/Hall sensor1/Subsystem ==
  theta : Inport
  Trigonometric Function : Trigonometry  Operator=sincos
  Trigonometric Function2 : Trigonometry  Operator=atan2
  mech->elec : Gain
  rad->deg : Gain  Gain=180/pi  SaturateOnIntegerOverflow=on  OutDataTypeStr=Inherit: Same as input  ParamDataTypeStr=Inherit: Same as input
  deg : Outport
  wires:
  Trigonometric Function2/1 -> rad->deg/1
  Trigonometric Function/1 -> Trigonometric Function2/1
  theta/1 -> mech->elec/1
  rad->deg/1 -> deg/1
  Trigonometric Function/2 -> Trigonometric Function2/2
  mech->elec/1 -> Trigonometric Function/1

== matlab function bldc_cImpl/Inverter Controller/EM Controller/MATLAB Function ==
  data: u input
function fcn(u)

disp(u);

== matlab function bldc_cImpl/Inverter Controller/Hall sensors/Clocked speed calc/MATLAB Function ==
  data: hallA input; w output; hallB input; hallC input
function w = estSpeed(hallA, hallB, hallC)
% estSpeed Returns w as a speed est from hall effect inputs [rad/s]

    CLOCK_COUNTS=100; % how many clock cycles to count ticks over
    CLOCK_FREQ = 10000; % How often this code is invoked [Hz]
    
    w = hallSensorSpeedCalc(hallA, hallB, hallC, CLOCK_COUNTS, CLOCK_FREQ);

end
